simulink model "OFDM_Rx_HW"  (R2020a)
settings: Solver=FixedStepDiscrete  StartTime=0.0  StopTime=inf  RelTol=1e-3
InitFcn:
  | % Set parameters
  | fs = 20e6;
  | fclk = 240e6;
  | ssr = 2;
  | fdc = fclk*ssr*8;
  | 
  | % Load libraries
  | addpath('./lib');
  | 
  | % Load all required variables
  | load('variables/read_addr_data');
  | load('variables/read_addr_cp');
  | load('variables/read_addr_pream');
  | load('variables/read_addr_rx');
  | load('variables/pilot');
  | load('variables/sc_index');
  | load('variables/LTSfreq');
  | load('variables/STSfreq');
  | load('variables/LTSread');
  | load('variables/STSread');
  | 
  | run ./scripts/rfgen;
undefined symbols (not defined in the file): LTSfreq, pilot, read_addr_rx, sc_index
libraries: simulink x36, hdlsllib x30, dsphdlmathfun x3, dspsigops x2, dsphdlxfrm x1, dsphdlsigops x1
(part 1 of 3)
settings Model: DataTypeOverride=Off  Creator=njb13206  LastModifiedBy=andy
settings OptimizationCC: BlockReduction=off  ConditionallyExecuteInputs=off  DefaultParameterBehavior=Inlined
settings DebuggingCC: AlgebraicLoopMsg=error  SingleTaskRateTransMsg=error  IntegerOverflowMsg=none  ParameterPrecisionLossMsg=none  IntegerSaturationMsg=none
settings HardwareCC: ProdBitPerPointer=32  ProdBitPerSizeT=32  ProdBitPerPtrDiffT=32  ProdLargestAtomicFloat=None  ProdIntDivRoundTo=Undefined  ProdEndianess=Unspecified  ProdWordSize=32  ProdHWDeviceType=ASIC/FPGA->ASIC/FPGA  TargetBitPerLong=64  TargetBitPerPointer=64  TargetBitPerSizeT=64  TargetBitPerPtrDiffT=64  TargetLongLongMode=on  TargetIntDivRoundTo=Zero  TargetEndianess=LittleEndian  TargetWordSize=64  TargetHWDeviceType=Custom Processor->MATLAB Host Computer  ProdEqTarget=off

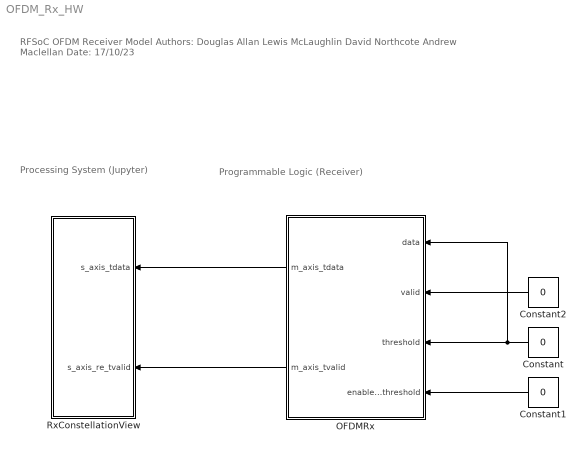
== system OFDM_Rx_HW ==
  note: Processing System (Jupyter)
  note: RFSoC OFDM Receiver Model
      | Authors: Douglas Allan
      | Lewis McLaughlin
      | David Northcote
      | Andrew Maclellan
      | Date: 17/10/23
  note: Programmable Logic (Receiver)
  Constant : Constant  Value=0  OutDataTypeStr=uint32  SampleTime=-1
  Constant1 : Constant  Value=0  OutDataTypeStr=uint32  SampleTime=-1
  Constant2 : Constant  Value=0  OutDataTypeStr=boolean  SampleTime=-1
  OFDMRx : Subsystem  TreatAsAtomicUnit=on
  RxConstellationView : Subsystem
  wires:
  OFDMRx/1(m_axis_tdata) -> RxConstellationView/1(s_axis_tdata)
  OFDMRx/2(m_axis_tvalid) -> RxConstellationView/2(s_axis_re_tvalid)
  Constant1/1 -> OFDMRx/4(enable_threshold)
  Constant/1 -> OFDMRx/3(threshold), OFDMRx/1(data)
  Constant2/1 -> OFDMRx/2(valid)

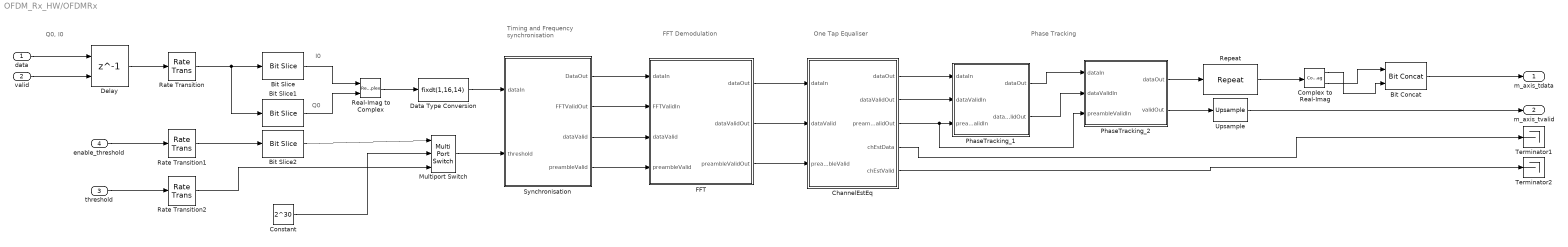
== system OFDM_Rx_HW/OFDMRx ==
  note: Phase Tracking
  note: One Tap Equaliser
  note: FFT Demodulation
  note: Timing and Frequency
      | synchronisation
  note: Q0, I0
  note: I0
  note: Q0
  data : Inport
  valid : Inport  Port=2
  threshold : Inport  Port=3
  enable_threshold : Inport  Port=4
  Bit Concat : hdlsllib/Logic and Bit Operations/Bit Concat  numInputs=2
  Bit Slice : hdlsllib/Logic and Bit Operations/Bit Slice  lidx=15  ridx=0
      settings: SourceProductBaseCode=SL
  Bit Slice1 : hdlsllib/Logic and Bit Operations/Bit Slice  lidx=31  ridx=16
      settings: SourceProductBaseCode=SL
  Bit Slice2 : hdlsllib/Logic and Bit Operations/Bit Slice  lidx=0  ridx=0
      settings: SourceProductBaseCode=SL
  ChannelEstEq : Subsystem
  Complex to Real-Imag : ComplexToRealImag
  Constant : Constant  Value=2^30  OutDataTypeStr=uint32  SampleTime=-1
  Data Type Conversion : DataTypeConversion  OutDataTypeStr=fixdt(1,16,14)  ConvertRealWorld=Stored Integer (SI)
  Delay : Delay  DelayLength=1  ShowEnablePort=on
      settings: InputPortMap=u0,e6
  FFT : Subsystem
  Multiport Switch : MultiPortSwitch  DataPortOrder=Zero-based contiguous  Inputs=2  zeroidx=on
  PhaseTracking_1 : Subsystem
  PhaseTracking_2 : Subsystem
  Rate Transition : RateTransition  OutPortSampleTime=1/fs
  Rate Transition1 : RateTransition  OutPortSampleTime=1/fs
  Rate Transition2 : RateTransition  OutPortSampleTime=1/fs
  Real-Imag to Complex : RealImagToComplex
  Repeat : dspsigops/Repeat  N=12  InputProcessing=Columns as channels (frame based)  RateOptions=Allow multirate processing  ic=0  mode=Unused parameter value
  Synchronisation : Subsystem
  Terminator1 : Terminator
  Terminator2 : Terminator
  Upsample : dspsigops/Upsample  N=12  phase=5  RateOptions=Allow multirate processing  ic=0  mode=Unused parameter value
  m_axis_tdata : Outport  VectorParamsAs1DForOutWhenUnconnected=off
  m_axis_tvalid : Outport  Port=2  VectorParamsAs1DForOutWhenUnconnected=off
  wires:
  valid/1 -> Delay/2
  Bit Slice1/1 -> Real-Imag to Complex/2
  Bit Slice/1 -> Real-Imag to Complex/1
  Complex to Real-Imag/1 -> Bit Concat/2
  Complex to Real-Imag/2 -> Bit Concat/1
  Repeat/1 -> Complex to Real-Imag/1
  PhaseTracking_2/2(validOut) -> Upsample/1
  PhaseTracking_2/1(dataOut) -> Repeat/1
  Data Type Conversion/1 -> Synchronisation/1(dataIn)
  Real-Imag to Complex/1 -> Data Type Conversion/1
  FFT/1(dataOut) -> ChannelEstEq/1(dataIn)
  FFT/3(preambleValidOut) -> ChannelEstEq/3(preambleValid)
  FFT/2(dataValidOut) -> ChannelEstEq/2(dataValid)
  Synchronisation/1(DataOut) -> FFT/1(dataIn)
  Synchronisation/2(FFTValidOut) -> FFT/2(FFTValidIn)
  Synchronisation/3(dataValid) -> FFT/3(dataValid)
  Synchronisation/4(preambleValid) -> FFT/4(preambleValid)
  ChannelEstEq/1(dataOut) -> PhaseTracking_1/1(dataIn)
  ChannelEstEq/2(dataValidOut) -> PhaseTracking_1/2(dataValidIn)
  PhaseTracking_1/1(dataOut) -> PhaseTracking_2/1(dataIn)
  PhaseTracking_1/2(dataValidOut) -> PhaseTracking_2/2(dataValidIn)
  ChannelEstEq/5(chEstValid) -> Terminator2/1
  ChannelEstEq/4(chEstData) -> Terminator1/1
  Multiport Switch/1 -> Synchronisation/2(threshold)
  threshold/1 -> Rate Transition2/1
  Constant/1 -> Multiport Switch/2
  enable_threshold/1 -> Rate Transition1/1
  Bit Concat/1 -> m_axis_tdata/1
  Upsample/1 -> m_axis_tvalid/1
  Bit Slice2/1 -> Multiport Switch/1
  Rate Transition/1 -> Bit Slice/1, Bit Slice1/1
  Rate Transition1/1 -> Bit Slice2/1
  Rate Transition2/1 -> Multiport Switch/3
  Delay/1 -> Rate Transition/1
  data/1 -> Delay/1
  ChannelEstEq/3(preambleValidOut) -> PhaseTracking_2/3(preambleValidIn), PhaseTracking_1/3(preambleValidIn)

== system OFDM_Rx_HW/RxConstellationView ==
  s_axis_tdata : Inport
  s_axis_re_tvalid : Inport  Port=2
  Bit Slice : hdlsllib/Logic and Bit Operations/Bit Slice  lidx=15  ridx=0
      settings: SourceProductBaseCode=SL
  Bit Slice1 : hdlsllib/Logic and Bit Operations/Bit Slice  lidx=31  ridx=16
      settings: SourceProductBaseCode=SL
  Constant : Constant  Value=NaN + 1i*NaN  OutDataTypeStr=double  SampleTime=-1
  Constellation Diagram : ConstellationDiagram
  Data Type Conversion : DataTypeConversion  OutDataTypeStr=fixdt(1,16,14)  ConvertRealWorld=Stored Integer (SI)
  Real-Imag to Complex : RealImagToComplex
  Switch : Switch  Criteria=u2 ~= 0
  wires:
  Switch/1 -> Constellation Diagram/1
  Constant/1 -> Switch/3
  s_axis_re_tvalid/1 -> Switch/2
  Real-Imag to Complex/1 -> Data Type Conversion/1
  Bit Slice/1 -> Real-Imag to Complex/1
  s_axis_tdata/1 -> Bit Slice1/1, Bit Slice/1
  Bit Slice1/1 -> Real-Imag to Complex/2
  Data Type Conversion/1 -> Switch/1

== system OFDM_Rx_HW/OFDMRx/ChannelEstEq ==
  dataIn : Inport
  dataValid : Inport  Port=2
  preambleValid : Inport  Port=3
  Bit Concat1 : hdlsllib/Logic and Bit Operations/Bit Concat  numInputs=2
  ChannelEstimate : Subsystem
  Complex to Real-Imag1 : ComplexToRealImag
  Data Type Conversion1 : DataTypeConversion  OutDataTypeStr=fixdt(1,16,14)
  Data Type Conversion3 : DataTypeConversion  OutDataTypeStr=uint16  ConvertRealWorld=Stored Integer (SI)
  Data Type Conversion4 : DataTypeConversion  OutDataTypeStr=uint16  ConvertRealWorld=Stored Integer (SI)
  Delay : Delay  DelayLength=6
  Delay1 : Delay  DelayLength=6
  Delay2 : Delay  DelayLength=5
  Equalise : Subsystem
  dataOut : Outport  VectorParamsAs1DForOutWhenUnconnected=off
  dataValidOut : Outport  Port=2  VectorParamsAs1DForOutWhenUnconnected=off
  preambleValidOut : Outport  Port=3  VectorParamsAs1DForOutWhenUnconnected=off
  chEstData : Outport  Port=4  VectorParamsAs1DForOutWhenUnconnected=off
  chEstValid : Outport  Port=5  VectorParamsAs1DForOutWhenUnconnected=off
  wires:
  ChannelEstimate/1(chEstOut) -> Equalise/2(chEstIn), Data Type Conversion1/1
  Delay/1 -> Equalise/1(dataInEq)
  dataIn/1 -> ChannelEstimate/1(dataIn), Delay/1
  preambleValid/1 -> Delay1/1, ChannelEstimate/2(preambleValid)
  dataValid/1 -> ChannelEstimate/3(dataValidIn)
  Equalise/1(dataOutEq) -> dataOut/1
  Equalise/2(dataValidOut) -> dataValidOut/1
  ChannelEstimate/2(dataValidOut) -> chEstValid/1, Equalise/3(dataValidIn)
  Data Type Conversion4/1 -> Bit Concat1/1
  Bit Concat1/1 -> chEstData/1
  Data Type Conversion3/1 -> Bit Concat1/2
  Complex to Real-Imag1/2 -> Data Type Conversion4/1
  Complex to Real-Imag1/1 -> Data Type Conversion3/1
  Data Type Conversion1/1 -> Complex to Real-Imag1/1
  Delay1/1 -> Delay2/1
  Delay2/1 -> preambleValidOut/1

== system OFDM_Rx_HW/OFDMRx/FFT ==
  dataIn : Inport
  FFTValidIn : Inport  Port=2
  dataValid : Inport  Port=3
  preambleValid : Inport  Port=4
  Delay1 : Delay  DelayLength=173
  Delay2 : Delay  DelayLength=173
  FFT HDL Optimized : dsphdlxfrm/FFT HDL Optimized  FFTLength=64  Architecture=Streaming Radix 2^2  ComplexMultiplication=Use 4 multipliers and 2 adders  BitReversedOutput=off  BitReversedInput=off  Normalize=off  SimulateUsing=Code generation  RoundingMethod=Floor  ResetInputPort=off  StartOutputPort=off  EndOutputPort=off
      settings: SourceProductBaseCode=DS
  Terminator : Terminator
  dataOut : Outport  VectorParamsAs1DForOutWhenUnconnected=off
  dataValidOut : Outport  Port=2  VectorParamsAs1DForOutWhenUnconnected=off
  preambleValidOut : Outport  Port=3  VectorParamsAs1DForOutWhenUnconnected=off
  wires:
  FFTValidIn/1 -> FFT HDL Optimized/2
  dataIn/1 -> FFT HDL Optimized/1
  Delay2/1 -> dataValidOut/1
  Delay1/1 -> preambleValidOut/1
  FFT HDL Optimized/1 -> dataOut/1
  FFT HDL Optimized/2 -> Terminator/1
  dataValid/1 -> Delay2/1
  preambleValid/1 -> Delay1/1

== system OFDM_Rx_HW/OFDMRx/PhaseTracking_1 ==
  note: Phase Tracking Stage 1: Track linear phase error which occurs due to sampling phase/frequency offsets. The implemented algorithm
      | estimates the gradient of the linear phase error using pilot sub-carriers.
  dataIn : Inport
  dataValidIn : Inport  Port=2
  preambleValidIn : Inport  Port=3
  CordicRotate : Subsystem
  DataArrange : Subsystem
  "GradientEstimate " : Subsystem
  PhaseErrorEst : Subsystem
  PilotCtrlGen : Subsystem
  dataOut : Outport
  dataValidOut : Outport  Port=2
  wires:
  CordicRotate/2(dataValidOut) -> dataValidOut/1
  PhaseErrorEst/3(dataValidOut) -> CordicRotate/3(dataValidIn)
  PhaseErrorEst/2(PhaseOut) -> CordicRotate/2(PhaseInRotate)
  PhaseErrorEst/1(dataOut) -> CordicRotate/1(DataInRotate)
  "GradientEstimate "/1(dataOut) -> PhaseErrorEst/1(dataIn)
  "GradientEstimate "/2(gradientOut) -> PhaseErrorEst/2(gradientIn)
  "GradientEstimate "/3(dataValidOut) -> PhaseErrorEst/3(dataValidIn)
  CordicRotate/1("DataOutRotate  ") -> dataOut/1
  dataIn/1 -> DataArrange/1(dataIn)
  dataValidIn/1 -> DataArrange/2(dataValidIn)
  DataArrange/1(dataOut) -> PilotCtrlGen/1(dataIn)
  DataArrange/2(dataValidOut) -> PilotCtrlGen/2(validIn)
  PilotCtrlGen/1(dataOut) -> "GradientEstimate "/1(dataIn)
  PilotCtrlGen/2(pilotOut) -> "GradientEstimate "/2(pilotIn)
  PilotCtrlGen/3(pilotEnd) -> "GradientEstimate "/3(PilotEnd)
  PilotCtrlGen/4(dataValid) -> "GradientEstimate "/4(dataValid)
  DataArrange/3(frameDetOut) -> PilotCtrlGen/3(preambleValidIn)
  preambleValidIn/1 -> DataArrange/3(preambleValidIn)

== system OFDM_Rx_HW/OFDMRx/PhaseTracking_2 ==
  note: Phase Tracking Stage 2:  Track Common Phase Error (CPE) from symbol to symbol.
      | CPE is caused by residual frequency offset and phase noise effects.
  dataIn : Inport
  dataValidIn : Inport  Port=2
  preambleValidIn : Inport  Port=3
  CordicRotate : Subsystem
  PhaseEst : Subsystem
  PilotCtrlGen : Subsystem
  dataOut : Outport  VectorParamsAs1DForOutWhenUnconnected=off
  validOut : Outport  Port=2  VectorParamsAs1DForOutWhenUnconnected=off
  wires:
  PilotCtrlGen/1(dataOut) -> PhaseEst/1(dataIn)
  PilotCtrlGen/2(pilotOut) -> PhaseEst/2(PilotIn)
  PilotCtrlGen/3(PilotEnd) -> PhaseEst/3(pilotEnd)
  PilotCtrlGen/4(dataValid) -> PhaseEst/4(dataValid)
  PhaseEst/1(dataOut) -> CordicRotate/1(DataIn)
  PhaseEst/2(phaseOut) -> CordicRotate/2(PhaseIn)
  PhaseEst/3(validOut) -> CordicRotate/3(validIn)
  CordicRotate/1("DataOut  ") -> dataOut/1
  CordicRotate/2(validOut) -> validOut/1
  dataIn/1 -> PilotCtrlGen/1(dataIn)
  dataValidIn/1 -> PilotCtrlGen/2(ValidIn)
  preambleValidIn/1 -> PilotCtrlGen/3(preambleValidIn)

== system OFDM_Rx_HW/OFDMRx/Synchronisation ==
  dataIn : Inport
  threshold : Inport  Port=2
  CoarseFreqCorr : Subsystem
  ControlSigGen : Subsystem
  Delay : Subsystem
  Delay1 : Delay  DelayLength=22  InputProcessing=Columns as channels (frame based)
  Delay2 : Delay  InputProcessing=Columns as channels (frame based)
  Delay4 : Delay  DelayLength=1  InputProcessing=Columns as channels (frame based)
  FrameDetect : Subsystem
  "SchmidlCoxMetric " : Subsystem
  DataOut : Outport  VectorParamsAs1DForOutWhenUnconnected=off
  FFTValidOut : Outport  Port=2  VectorParamsAs1DForOutWhenUnconnected=off
  dataValid : Outport  Port=3  VectorParamsAs1DForOutWhenUnconnected=off
  preambleValid : Outport  Port=4  VectorParamsAs1DForOutWhenUnconnected=off
  wires:
  dataIn/1 -> "SchmidlCoxMetric "/1(dataIn), Delay1/1
  ControlSigGen/1(FFTValid) -> FFTValidOut/1
  ControlSigGen/2(dataValid) -> dataValid/1
  ControlSigGen/3(preambleValid) -> preambleValid/1  "preamble"
  Delay1/1 -> Delay2/1
  "SchmidlCoxMetric "/1(left) -> FrameDetect/1(leftIn)
  "SchmidlCoxMetric "/2(right) -> FrameDetect/2(rightIn)
  "SchmidlCoxMetric "/3(phase) -> FrameDetect/3(phaseIn)
  FrameDetect/2(phaseOut) -> CoarseFreqCorr/3(phaseIn)
  Delay2/1 -> CoarseFreqCorr/1(dataIn)
  FrameDetect/1(frameDet) -> CoarseFreqCorr/2(frameDet)
  Delay4/1 -> DataOut/1
  CoarseFreqCorr/2(frameDetOut) -> Delay/2(strobe)
  CoarseFreqCorr/1(dataOut) -> Delay/1(data)
  Delay/2(strobeOut) -> ControlSigGen/1(validIn)
  Delay/1(dataOut) -> Delay4/1
  threshold/1 -> "SchmidlCoxMetric "/2(threshold)

== system OFDM_Rx_HW/OFDMRx/ChannelEstEq/ChannelEstimate ==
  note: Note the preamble symbols do not pass this point.
  note: Write averaged channel estimate to RAM and read out when data is valid
      | for equalisation of successive OFDM symbols.
  note: Get and store the channel estimate using the two
      | repetitions of the L-LTF
  dataIn : Inport
  preambleValid : Inport  Port=2
  dataValidIn : Inport  Port=3
  ChanEst : Subsystem
  Delay : Delay  DelayLength=5
  Delay1 : Delay  DelayLength=5
  Delay2 : Delay  DelayLength=1
  Dual Port RAM1 : hdlsllib/HDL RAMs/Dual Port RAM  ram_size=6
      settings: SourceProductBaseCode=SL
  HDL Counter3 : hdlsllib/Sources/HDL Counter  CountType=Count limited  CountInit=0  CountStep=1  CountMax=63  CountFromType=Initial value  CountFrom=0  CountResetPort=off  CountLoadPort=off  CountEnbPort=on  CountDirPort=off  CountDataType=Unsigned  CountWordLen=6  CountFracLen=0  CountSampTime=1
  Terminator : Terminator
  WriteEnbAddrGen : Subsystem
  chEstOut : Outport  VectorParamsAs1DForOutWhenUnconnected=off
  dataValidOut : Outport  Port=2  VectorParamsAs1DForOutWhenUnconnected=off
  wires:
  HDL Counter3/1 -> Dual Port RAM1/4
  Dual Port RAM1/2 -> chEstOut/1
  Delay2/1 -> dataValidOut/1
  preambleValid/1 -> ChanEst/2(PreambValidIn), Delay/1
  dataIn/1 -> ChanEst/1(ChanEstIn)
  ChanEst/1(ChEstOut) -> Dual Port RAM1/1
  dataValidIn/1 -> Delay1/1
  Delay1/1 -> HDL Counter3/1, Delay2/1
  Delay/1 -> WriteEnbAddrGen/1(In1)
  WriteEnbAddrGen/1(Out1) -> Dual Port RAM1/2
  WriteEnbAddrGen/2(Out2) -> Dual Port RAM1/3
  Dual Port RAM1/1 -> Terminator/1

== system OFDM_Rx_HW/OFDMRx/ChannelEstEq/Equalise ==
  note: Perform a complex division to obtain equalised data symbols.
  dataInEq : Inport
  chEstIn : Inport  Port=2
  dataValidIn : Inport  Port=3
  Abs2 : Subsystem
  Complex Mult : Subsystem
  Delay1 : Delay
  Delay8 : Delay  DelayLength=3
  Divide : Subsystem
  dataOutEq : Outport  VectorParamsAs1DForOutWhenUnconnected=off
  dataValidOut : Outport  Port=2  VectorParamsAs1DForOutWhenUnconnected=off
  wires:
  dataValidIn/1 -> Delay8/1
  chEstIn/1 -> Abs2/1(ChEstIn), Complex Mult/2(In2)
  dataInEq/1 -> Complex Mult/1(In1)
  Complex Mult/1(Out1) -> Divide/1(In1)
  Abs2/1(Out1) -> Divide/2(In2)
  Delay8/1 -> Delay1/1
  Delay1/1 -> dataValidOut/1
  Divide/1(dataOutEq) -> dataOutEq/1

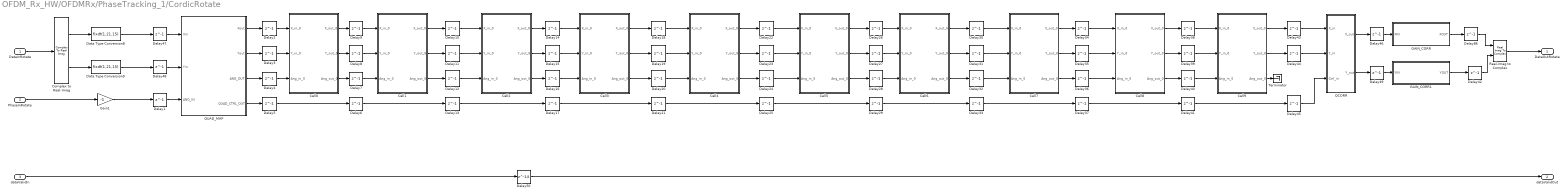
== system OFDM_Rx_HW/OFDMRx/PhaseTracking_1/CordicRotate ==
  DataInRotate : Inport
  PhaseInRotate : Inport  Port=2
  dataValidIn : Inport  Port=3
  Cell0 : Subsystem
  Cell1 : Subsystem
  Cell2 : Subsystem
  Cell3 : Subsystem
  Cell4 : Subsystem
  Cell5 : Subsystem
  Cell6 : Subsystem
  Cell7 : Subsystem
  Cell8 : Subsystem
  Cell9 : Subsystem
  Complex to Real-Imag : ComplexToRealImag
  Data Type Conversion8 : DataTypeConversion  OutDataTypeStr=fixdt(1,21,15)
  Data Type Conversion9 : DataTypeConversion  OutDataTypeStr=fixdt(1,21,15)
  Delay{1..49,86} (50 alike) : Delay  DelayLength=1
  Delay50 : Delay  DelayLength=14
  GAIN_CORR : Subsystem
  GAIN_CORR1 : Subsystem
  Gain1 : Gain  Gain=-1  OutDataTypeStr=fixdt(1,23,20)
  QCORR : Subsystem
  QUAD_MAP : Subsystem
  Real-Imag to Complex : RealImagToComplex
  Terminator : Terminator
  "DataOutRotate  " : Outport  VectorParamsAs1DForOutWhenUnconnected=off
  dataValidOut : Outport  Port=2  VectorParamsAs1DForOutWhenUnconnected=off
  wires:
  Delay50/1 -> dataValidOut/1
  dataValidIn/1 -> Delay50/1
  Gain1/1 -> Delay1/1
  PhaseInRotate/1 -> Gain1/1
  QCORR/1(X_out) -> Delay46/1
  Data Type Conversion9/1 -> Delay48/1
  Data Type Conversion8/1 -> Delay47/1
  Delay45/1 -> QCORR/3(Ctrl_in)
  Delay4/1 -> Cell0/3(Ang_in_0)
  Delay1/1 -> QUAD_MAP/3(ANG_IN)
  QCORR/2(Y_out) -> Delay49/1
  Delay49/1 -> GAIN_CORR1/1(YIN)
  Delay46/1 -> GAIN_CORR/1(XIN)
  Delay44/1 -> QCORR/2(Y_in)
  Delay43/1 -> QCORR/1(X_in)
  Cell9/2(Y_out_0) -> Delay44/1
  Cell9/1(X_out_0) -> Delay43/1
  Delay41/1 -> Delay45/1
  Cell9/3(Ang_out_0) -> Terminator/1
  GAIN_CORR1/1(YOUT) -> Delay42/1
  Cell8/1(X_out_0) -> Delay38/1
  Cell8/2(Y_out_0) -> Delay39/1
  Cell8/3(Ang_out_0) -> Delay40/1
  Delay37/1 -> Delay41/1
  Delay38/1 -> Cell9/1(X_in_0)
  Delay39/1 -> Cell9/2(Y_in_0)
  Delay40/1 -> Cell9/3(Ang_in_0)
  Delay36/1 -> Cell8/3(Ang_in_0)
  Delay35/1 -> Cell8/2(Y_in_0)
  Delay34/1 -> Cell8/1(X_in_0)
  Delay33/1 -> Delay37/1
  Cell7/3(Ang_out_0) -> Delay36/1
  Cell7/2(Y_out_0) -> Delay35/1
  Cell7/1(X_out_0) -> Delay34/1
  Cell6/1(X_out_0) -> Delay30/1
  Cell6/2(Y_out_0) -> Delay31/1
  Cell6/3(Ang_out_0) -> Delay32/1
  Delay29/1 -> Delay33/1
  Delay30/1 -> Cell7/1(X_in_0)
  Delay31/1 -> Cell7/2(Y_in_0)
  Delay32/1 -> Cell7/3(Ang_in_0)
  Delay28/1 -> Cell6/3(Ang_in_0)
  Delay27/1 -> Cell6/2(Y_in_0)
  Delay26/1 -> Cell6/1(X_in_0)
  Delay25/1 -> Delay29/1
  Cell5/3(Ang_out_0) -> Delay28/1
  Cell5/2(Y_out_0) -> Delay27/1
  Cell5/1(X_out_0) -> Delay26/1
  Cell4/1(X_out_0) -> Delay22/1
  Cell4/2(Y_out_0) -> Delay23/1
  Cell4/3(Ang_out_0) -> Delay24/1
  Delay21/1 -> Delay25/1
  Delay22/1 -> Cell5/1(X_in_0)
  Delay23/1 -> Cell5/2(Y_in_0)
  Delay24/1 -> Cell5/3(Ang_in_0)
  Delay20/1 -> Cell4/3(Ang_in_0)
  Delay19/1 -> Cell4/2(Y_in_0)
  Delay18/1 -> Cell4/1(X_in_0)
  Delay17/1 -> Delay21/1
  Cell3/3(Ang_out_0) -> Delay20/1
  Cell3/2(Y_out_0) -> Delay19/1
  Cell3/1(X_out_0) -> Delay18/1
  Cell2/1(X_out_0) -> Delay14/1
  Cell2/2(Y_out_0) -> Delay15/1
  Cell2/3(Ang_out_0) -> Delay16/1
  Delay13/1 -> Delay17/1
  Delay14/1 -> Cell3/1(X_in_0)
  Delay15/1 -> Cell3/2(Y_in_0)
  Delay16/1 -> Cell3/3(Ang_in_0)
  Delay12/1 -> Cell2/3(Ang_in_0)
  Delay11/1 -> Cell2/2(Y_in_0)
  Delay10/1 -> Cell2/1(X_in_0)
  Delay6/1 -> Delay13/1
  Cell1/3(Ang_out_0) -> Delay12/1
  Cell1/2(Y_out_0) -> Delay11/1
  Cell1/1(X_out_0) -> Delay10/1
  Delay9/1 -> Cell1/1(X_in_0)
  Delay8/1 -> Cell1/2(Y_in_0)
  Delay7/1 -> Cell1/3(Ang_in_0)
  Delay5/1 -> Delay6/1
  Cell0/3(Ang_out_0) -> Delay7/1
  Cell0/2(Y_out_0) -> Delay8/1
  Cell0/1(X_out_0) -> Delay9/1
  QUAD_MAP/4(QUAD_CTRL_OUT) -> Delay5/1
  Delay3/1 -> Cell0/2(Y_in_0)
  Delay2/1 -> Cell0/1(X_in_0)
  QUAD_MAP/3(ANG_OUT) -> Delay4/1
  QUAD_MAP/2(Yout) -> Delay3/1
  QUAD_MAP/1(Xout) -> Delay2/1
  Delay47/1 -> QUAD_MAP/1(Xin)
  Delay48/1 -> QUAD_MAP/2(Yin)
  GAIN_CORR/1(XOUT) -> Delay86/1
  Complex to Real-Imag/2 -> Data Type Conversion9/1
  DataInRotate/1 -> Complex to Real-Imag/1
  Complex to Real-Imag/1 -> Data Type Conversion8/1
  Delay86/1 -> Real-Imag to Complex/1
  Delay42/1 -> Real-Imag to Complex/2
  Real-Imag to Complex/1 -> "DataOutRotate  "/1

== system OFDM_Rx_HW/OFDMRx/PhaseTracking_1/DataArrange ==
  note: Re-arrange data symbols
  dataIn : Inport
  dataValidIn : Inport  Port=2
  preambleValidIn : Inport  Port=3
  Delay : Delay  DelayLength=64  InitialCondition=0  UseCircularBuffer=on
  Delay1 : Delay  DelayLength=65
  Delay3 : Delay  DelayLength=1  InitialCondition=0  UseCircularBuffer=on
  Dual Port RAM : hdlsllib/HDL RAMs/Dual Port RAM  ram_size=7
      settings: SourceProductBaseCode=SL
  HDL Counter : hdlsllib/Sources/HDL Counter  CountType=Count limited  CountInit=0  CountStep=1  CountMax=127  CountFromType=Initial value  CountFrom=0  CountResetPort=off  CountLoadPort=off  CountEnbPort=on  CountDirPort=off  CountDataType=Unsigned  CountWordLen=7  CountFracLen=0  CountSampTime=1
  HDL Counter1 : hdlsllib/Sources/HDL Counter  CountType=Count limited  CountInit=0  CountStep=1  CountMax=127  CountFromType=Initial value  CountFrom=0  CountResetPort=off  CountLoadPort=off  CountEnbPort=on  CountDirPort=off  CountDataType=Unsigned  CountWordLen=7  CountFracLen=0  CountSampTime=1
  READ_ADDRESS : Lookup_n-D  NumberOfTableDimensions=1  LookupTableObject=''  BreakpointsForDimension1=[0:127]  BreakpointsForDimension1FirstPoint=10  BreakpointsForDimension2FirstPoint=10  BreakpointsForDimension1Spacing=12  BreakpointsForDimension2Spacing=12  IndexSearchMethod=Evenly spaced points  Table=read_addr_rx  TableDataTypeStr=fixdt(0,7,0)  InterpMethod=Flat  DiagnosticForOutOfRangeInput=Error  InternalRulePriority=Speed  OutDataTypeStr=fixdt(0,7,0)  RndMeth=Simplest  InputSameDT=on
  READ_CTRL : Subsystem
  Terminator : Terminator
  dataValidGen : Subsystem
  dataOut : Outport  VectorParamsAs1DForOutWhenUnconnected=off
  dataValidOut : Outport  Port=2  VectorParamsAs1DForOutWhenUnconnected=off
  frameDetOut : Outport  Port=3  VectorParamsAs1DForOutWhenUnconnected=off
  wires:
  Dual Port RAM/1 -> Terminator/1
  dataValidIn/1 -> Delay/1, HDL Counter1/1, Dual Port RAM/3
  HDL Counter/1 -> READ_ADDRESS/1
  Dual Port RAM/2 -> dataOut/1
  dataIn/1 -> Dual Port RAM/1
  HDL Counter1/1 -> Dual Port RAM/2
  Delay/1 -> HDL Counter/1, Delay3/1, READ_CTRL/2(In2)
  READ_CTRL/1(Out1) -> Dual Port RAM/4
  READ_ADDRESS/1 -> READ_CTRL/1(In1)
  Delay3/1 -> dataValidGen/1(enb)
  dataValidGen/1(dataValidOut) -> dataValidOut/1
  Delay1/1 -> frameDetOut/1
  preambleValidIn/1 -> Delay1/1

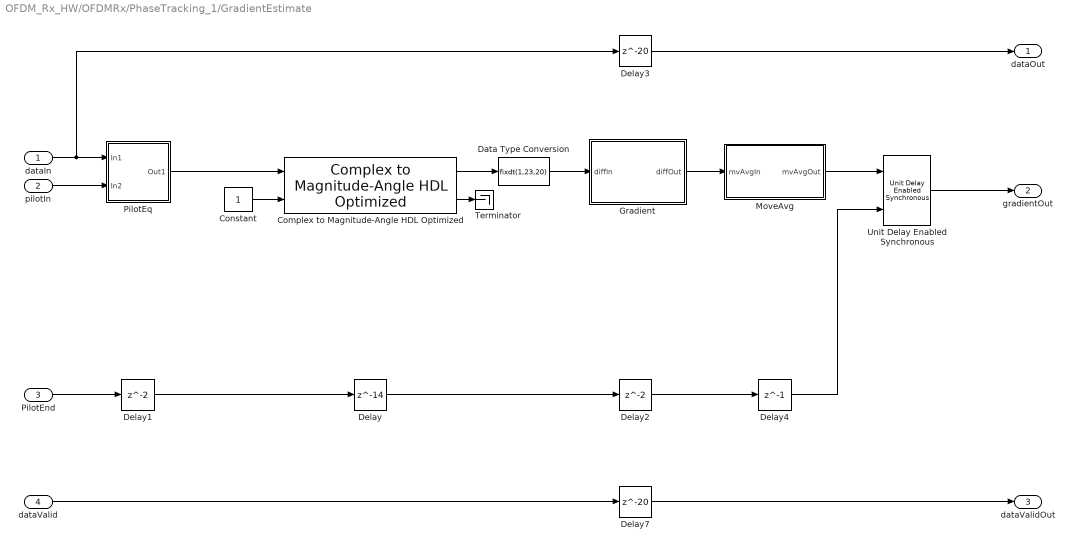
== system OFDM_Rx_HW/OFDMRx/PhaseTracking_1/GradientEstimate  ==
  dataIn : Inport
  pilotIn : Inport  Port=2
  PilotEnd : Inport  Port=3
  dataValid : Inport  Port=4
  Complex to Magnitude-Angle HDL Optimized : dsphdlmathfun/Complex to Magnitude-Angle HDL Optimized  NumIterationsSource=Property  NumIterations=10  OutputFormat=Angle  AngleFormat=Radians  ScaleOutput=off  SimulateUsing=Code generation
      settings: SourceProductBaseCode=DS
  Constant : Constant  OutDataTypeStr=boolean  SampleTime=1/fs
  Data Type Conversion : DataTypeConversion  OutDataTypeStr=fixdt(1,23,20)
  Delay : Delay  DelayLength=14
  Delay1 : Delay
  Delay2 : Delay
  Delay3 : Delay  DelayLength=20
  Delay4 : Delay  DelayLength=1
  Delay7 : Delay  DelayLength=20
  Gradient : Subsystem
  MoveAvg : Subsystem
  PilotEq : Subsystem
  Terminator : Terminator
  Unit Delay Enabled Synchronous : hdlsllib/Discrete/Unit Delay Enabled Synchronous  InitialCondition=0.0  SampleTime=-1
      settings: SourceProductBaseCode=SL
  dataOut : Outport  VectorParamsAs1DForOutWhenUnconnected=off
  gradientOut : Outport  Port=2  VectorParamsAs1DForOutWhenUnconnected=off
  dataValidOut : Outport  Port=3  VectorParamsAs1DForOutWhenUnconnected=off
  wires:
  Delay2/1 -> Delay4/1
  Data Type Conversion/1 -> Gradient/1(diffIn)
  Complex to Magnitude-Angle HDL Optimized/2 -> Terminator/1
  Constant/1 -> Complex to Magnitude-Angle HDL Optimized/2
  Complex to Magnitude-Angle HDL Optimized/1 -> Data Type Conversion/1
  Delay7/1 -> dataValidOut/1
  Unit Delay Enabled Synchronous/1 -> gradientOut/1
  Delay3/1 -> dataOut/1
  MoveAvg/1(mvAvgOut) -> Unit Delay Enabled Synchronous/1
  Delay1/1 -> Delay/1
  PilotEq/1(Out1) -> Complex to Magnitude-Angle HDL Optimized/1
  pilotIn/1 -> PilotEq/2(In2)
  dataIn/1 -> PilotEq/1(In1), Delay3/1
  Gradient/1(diffOut) -> MoveAvg/1(mvAvgIn)
  dataValid/1 -> Delay7/1
  PilotEnd/1 -> Delay1/1
  Delay/1 -> Delay2/1
  Delay4/1 -> Unit Delay Enabled Synchronous/2

== system OFDM_Rx_HW/OFDMRx/PhaseTracking_1/PhaseErrorEst ==
  dataIn : Inport
  gradientIn : Inport  Port=2
  dataValidIn : Inport  Port=3
  Delay{2..8} (7 alike) : Delay  DelayLength=1
  HDL Counter : hdlsllib/Sources/HDL Counter  CountType=Count limited  CountInit=0  CountStep=1  CountMax=51  CountFromType=Initial value  CountFrom=0  CountResetPort=on  CountLoadPort=off  CountEnbPort=on  CountDirPort=off  CountDataType=Unsigned  CountWordLen=6  CountFracLen=0  CountSampTime=1
  LUT : Lookup_n-D  NumberOfTableDimensions=1  BreakpointsForDimension1=0:51  IndexSearchMethod=Evenly spaced points  Table=sc_index  TableDataTypeStr=fixdt(1,6,0)  InterpMethod=Flat  ExtrapMethod=Clip  DiagnosticForOutOfRangeInput=Error  UseLastTableValue=on  InternalRulePriority=Speed  OutDataTypeStr=fixdt(1,6,0)  RndMeth=Simplest  InputSameDT=on
  NOT : Logic  Operator=NOT  IconShape=distinctive  AllPortsSameDT=off  OutDataTypeStr=boolean
  Product : Product  OutDataTypeStr=fixdt(1,23,20)
  dataOut : Outport  VectorParamsAs1DForOutWhenUnconnected=off
  PhaseOut : Outport  Port=2  VectorParamsAs1DForOutWhenUnconnected=off
  dataValidOut : Outport  Port=3  VectorParamsAs1DForOutWhenUnconnected=off
  wires:
  Delay8/1 -> dataValidOut/1
  Delay4/1 -> Delay8/1
  Delay7/1 -> PhaseOut/1
  Product/1 -> Delay7/1
  Delay6/1 -> dataOut/1
  Delay2/1 -> Delay6/1
  Delay5/1 -> Product/2
  Delay3/1 -> Product/1
  HDL Counter/1 -> LUT/1
  NOT/1 -> HDL Counter/1
  LUT/1 -> Delay5/1
  gradientIn/1 -> Delay3/1
  dataIn/1 -> Delay2/1
  dataValidIn/1 -> HDL Counter/2, Delay4/1, NOT/1

== system OFDM_Rx_HW/OFDMRx/PhaseTracking_1/PilotCtrlGen ==
  dataIn : Inport
  validIn : Inport  Port=2
  preambleValidIn : Inport  Port=3
  CtrlSigGen : Subsystem
  Delay1 : Delay  DelayLength=1
  Delay10 : Delay  DelayLength=1
  SampleCounter : Subsystem
  SymbolCounter : Subsystem
  pilotGen : Subsystem
  dataOut : Outport  VectorParamsAs1DForOutWhenUnconnected=off
  pilotOut : Outport  Port=2  VectorParamsAs1DForOutWhenUnconnected=off
  pilotEnd : Outport  Port=3  VectorParamsAs1DForOutWhenUnconnected=off
  dataValid : Outport  Port=4  VectorParamsAs1DForOutWhenUnconnected=off
  wires:
  dataIn/1 -> Delay10/1
  Delay10/1 -> dataOut/1
  pilotGen/1(pilOut) -> pilotOut/1
  validIn/1 -> SampleCounter/1(Valid_In), Delay1/1, SymbolCounter/1(ValidIn)
  SymbolCounter/1(Symbl_cnt) -> pilotGen/1(symbCount)
  CtrlSigGen/1(dataValid) -> dataValid/1
  CtrlSigGen/2(pilotEnd) -> pilotEnd/1
  SampleCounter/1(Sample_Cnt) -> CtrlSigGen/2(sampleCount), pilotGen/2(sampleCount)
  Delay1/1 -> CtrlSigGen/1(valid), pilotGen/3(valid)
  preambleValidIn/1 -> SymbolCounter/2(preambleValidIn)

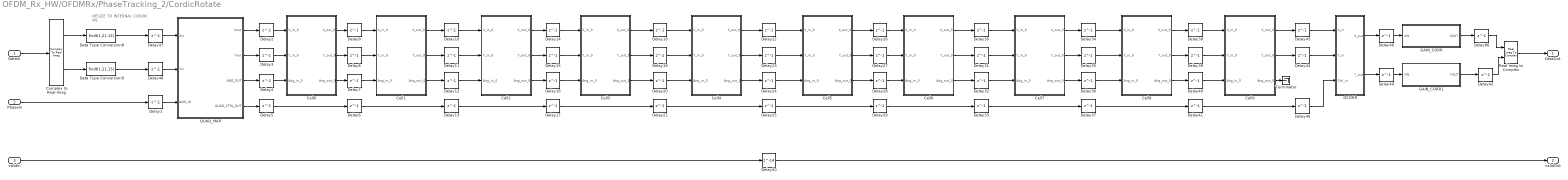
== system OFDM_Rx_HW/OFDMRx/PhaseTracking_2/CordicRotate ==
  note: RESIZE TO INTERNAL
      | CORDIC WL
  DataIn : Inport
  PhaseIn : Inport  Port=2
  validIn : Inport  Port=3
  Cell0 : Subsystem
  Cell1 : Subsystem
  Cell2 : Subsystem
  Cell3 : Subsystem
  Cell4 : Subsystem
  Cell5 : Subsystem
  Cell6 : Subsystem
  Cell7 : Subsystem
  Cell8 : Subsystem
  Cell9 : Subsystem
  Complex to Real-Imag : ComplexToRealImag
  Data Type Conversion8 : DataTypeConversion  OutDataTypeStr=fixdt(1,21,15)
  Data Type Conversion9 : DataTypeConversion  OutDataTypeStr=fixdt(1,21,15)
  Delay{1..49,86} (50 alike) : Delay  DelayLength=1
  Delay50 : Delay  DelayLength=14
  GAIN_CORR : Subsystem
  GAIN_CORR1 : Subsystem
  QCORR : Subsystem
  QUAD_MAP : Subsystem
  Real-Imag to Complex : RealImagToComplex
  Terminator : Terminator
  "DataOut  " : Outport  VectorParamsAs1DForOutWhenUnconnected=off
  validOut : Outport  Port=2  VectorParamsAs1DForOutWhenUnconnected=off
  wires:
  QCORR/1(X_out) -> Delay46/1
  PhaseIn/1 -> Delay1/1
  Data Type Conversion9/1 -> Delay48/1
  Data Type Conversion8/1 -> Delay47/1
  Delay45/1 -> QCORR/3(Ctrl_in)
  Delay4/1 -> Cell0/3(Ang_in_0)
  Delay1/1 -> QUAD_MAP/3(ANG_IN)
  QCORR/2(Y_out) -> Delay49/1
  Delay49/1 -> GAIN_CORR1/1(YIN)
  Delay46/1 -> GAIN_CORR/1(XIN)
  Delay44/1 -> QCORR/2(Y_in)
  Delay43/1 -> QCORR/1(X_in)
  Cell9/2(Y_out_0) -> Delay44/1
  Cell9/1(X_out_0) -> Delay43/1
  Delay41/1 -> Delay45/1
  Cell9/3(Ang_out_0) -> Terminator/1
  GAIN_CORR1/1(YOUT) -> Delay42/1
  Cell8/1(X_out_0) -> Delay38/1
  Cell8/2(Y_out_0) -> Delay39/1
  Cell8/3(Ang_out_0) -> Delay40/1
  Delay37/1 -> Delay41/1
  Delay38/1 -> Cell9/1(X_in_0)
  Delay39/1 -> Cell9/2(Y_in_0)
  Delay40/1 -> Cell9/3(Ang_in_0)
  Delay36/1 -> Cell8/3(Ang_in_0)
  Delay35/1 -> Cell8/2(Y_in_0)
  Delay34/1 -> Cell8/1(X_in_0)
  Delay33/1 -> Delay37/1
  Cell7/3(Ang_out_0) -> Delay36/1
  Cell7/2(Y_out_0) -> Delay35/1
  Cell7/1(X_out_0) -> Delay34/1
  Cell6/1(X_out_0) -> Delay30/1
  Cell6/2(Y_out_0) -> Delay31/1
  Cell6/3(Ang_out_0) -> Delay32/1
  Delay29/1 -> Delay33/1
  Delay30/1 -> Cell7/1(X_in_0)
  Delay31/1 -> Cell7/2(Y_in_0)
  Delay32/1 -> Cell7/3(Ang_in_0)
  Delay28/1 -> Cell6/3(Ang_in_0)
  Delay27/1 -> Cell6/2(Y_in_0)
  Delay26/1 -> Cell6/1(X_in_0)
  Delay25/1 -> Delay29/1
  Cell5/3(Ang_out_0) -> Delay28/1
  Cell5/2(Y_out_0) -> Delay27/1
  Cell5/1(X_out_0) -> Delay26/1
  Cell4/1(X_out_0) -> Delay22/1
  Cell4/2(Y_out_0) -> Delay23/1
  Cell4/3(Ang_out_0) -> Delay24/1
  Delay21/1 -> Delay25/1
  Delay22/1 -> Cell5/1(X_in_0)
  Delay23/1 -> Cell5/2(Y_in_0)
  Delay24/1 -> Cell5/3(Ang_in_0)
  Delay20/1 -> Cell4/3(Ang_in_0)
  Delay19/1 -> Cell4/2(Y_in_0)
  Delay18/1 -> Cell4/1(X_in_0)
  Delay17/1 -> Delay21/1
  Cell3/3(Ang_out_0) -> Delay20/1
  Cell3/2(Y_out_0) -> Delay19/1
  Cell3/1(X_out_0) -> Delay18/1
  Cell2/1(X_out_0) -> Delay14/1
  Cell2/2(Y_out_0) -> Delay15/1
  Cell2/3(Ang_out_0) -> Delay16/1
  Delay13/1 -> Delay17/1
  Delay14/1 -> Cell3/1(X_in_0)
  Delay15/1 -> Cell3/2(Y_in_0)
  Delay16/1 -> Cell3/3(Ang_in_0)
  Delay12/1 -> Cell2/3(Ang_in_0)
  Delay11/1 -> Cell2/2(Y_in_0)
  Delay10/1 -> Cell2/1(X_in_0)
  Delay6/1 -> Delay13/1
  Cell1/3(Ang_out_0) -> Delay12/1
  Cell1/2(Y_out_0) -> Delay11/1
  Cell1/1(X_out_0) -> Delay10/1
  Delay9/1 -> Cell1/1(X_in_0)
  Delay8/1 -> Cell1/2(Y_in_0)
  Delay7/1 -> Cell1/3(Ang_in_0)
  Delay5/1 -> Delay6/1
  Cell0/3(Ang_out_0) -> Delay7/1
  Cell0/2(Y_out_0) -> Delay8/1
  Cell0/1(X_out_0) -> Delay9/1
  QUAD_MAP/4(QUAD_CTRL_OUT) -> Delay5/1
  Delay3/1 -> Cell0/2(Y_in_0)
  Delay2/1 -> Cell0/1(X_in_0)
  QUAD_MAP/3(ANG_OUT) -> Delay4/1
  QUAD_MAP/2(Yout) -> Delay3/1
  QUAD_MAP/1(Xout) -> Delay2/1
  Delay47/1 -> QUAD_MAP/1(Xin)
  Delay48/1 -> QUAD_MAP/2(Yin)
  GAIN_CORR/1(XOUT) -> Delay86/1
  Complex to Real-Imag/2 -> Data Type Conversion9/1
  DataIn/1 -> Complex to Real-Imag/1
  Complex to Real-Imag/1 -> Data Type Conversion8/1
  Delay86/1 -> Real-Imag to Complex/1
  Delay42/1 -> Real-Imag to Complex/2
  Real-Imag to Complex/1 -> "DataOut  "/1
  validIn/1 -> Delay50/1
  Delay50/1 -> validOut/1

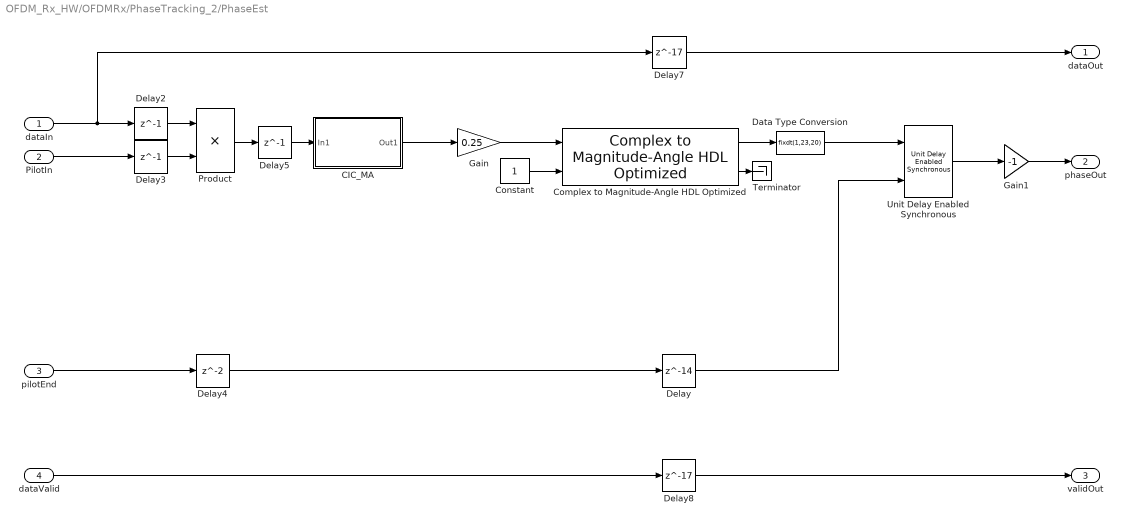
== system OFDM_Rx_HW/OFDMRx/PhaseTracking_2/PhaseEst ==
  dataIn : Inport
  PilotIn : Inport  Port=2
  pilotEnd : Inport  Port=3
  dataValid : Inport  Port=4
  CIC_MA : Subsystem
  Complex to Magnitude-Angle HDL Optimized : dsphdlmathfun/Complex to Magnitude-Angle HDL Optimized  NumIterationsSource=Property  NumIterations=10  OutputFormat=Angle  AngleFormat=Radians  ScaleOutput=off  SimulateUsing=Code generation
      settings: SourceProductBaseCode=DS
  Constant : Constant  OutDataTypeStr=boolean  SampleTime=1/fs
  Data Type Conversion : DataTypeConversion  OutDataTypeStr=fixdt(1,23,20)
  Delay : Delay  DelayLength=14
  Delay2 : Delay  DelayLength=1
  Delay3 : Delay  DelayLength=1
  Delay4 : Delay
  Delay5 : Delay  DelayLength=1
  Delay7 : Delay  DelayLength=17
  Delay8 : Delay  DelayLength=17
  Gain : Gain  Gain=0.25  OutDataTypeStr=fixdt(1,18,15)
  Gain1 : Gain  Gain=-1  OutDataTypeStr=fixdt(1,23,20)
  Product : Product  OutDataTypeStr=fixdt(1,18,15)
  Terminator : Terminator
  Unit Delay Enabled Synchronous : hdlsllib/Discrete/Unit Delay Enabled Synchronous  InitialCondition=0.0  SampleTime=-1
      settings: SourceProductBaseCode=SL
  dataOut : Outport  VectorParamsAs1DForOutWhenUnconnected=off
  phaseOut : Outport  Port=2  VectorParamsAs1DForOutWhenUnconnected=off
  validOut : Outport  Port=3  VectorParamsAs1DForOutWhenUnconnected=off
  wires:
  CIC_MA/1(Out1) -> Gain/1
  Delay/1 -> Unit Delay Enabled Synchronous/2
  PilotIn/1 -> Delay3/1
  dataIn/1 -> Delay7/1, Delay2/1
  Product/1 -> Delay5/1
  Delay2/1 -> Product/1
  Delay3/1 -> Product/2
  Delay5/1 -> CIC_MA/1(In1)
  pilotEnd/1 -> Delay4/1
  dataValid/1 -> Delay8/1
  Delay7/1 -> dataOut/1
  Unit Delay Enabled Synchronous/1 -> Gain1/1
  Delay8/1 -> validOut/1
  Constant/1 -> Complex to Magnitude-Angle HDL Optimized/2
  Gain/1 -> Complex to Magnitude-Angle HDL Optimized/1
  Complex to Magnitude-Angle HDL Optimized/1 -> Data Type Conversion/1
  Complex to Magnitude-Angle HDL Optimized/2 -> Terminator/1
  Delay4/1 -> Delay/1
  Gain1/1 -> phaseOut/1
  Data Type Conversion/1 -> Unit Delay Enabled Synchronous/1

== system OFDM_Rx_HW/OFDMRx/PhaseTracking_2/PilotCtrlGen ==
  dataIn : Inport
  ValidIn : Inport  Port=2
  preambleValidIn : Inport  Port=3
  CtrlSigGen : Subsystem
  Delay1 : Delay  DelayLength=1
  Delay10 : Delay  DelayLength=1
  SampleCounter : Subsystem
  SymbolCounter : Subsystem
  pilotGen : Subsystem
  dataOut : Outport  VectorParamsAs1DForOutWhenUnconnected=off
  pilotOut : Outport  Port=2  VectorParamsAs1DForOutWhenUnconnected=off
  PilotEnd : Outport  Port=3  VectorParamsAs1DForOutWhenUnconnected=off
  dataValid : Outport  Port=4  VectorParamsAs1DForOutWhenUnconnected=off
  wires:
  dataIn/1 -> Delay10/1
  Delay10/1 -> dataOut/1
  pilotGen/1(pilOut) -> pilotOut/1
  ValidIn/1 -> Delay1/1, SampleCounter/1(Valid_In), SymbolCounter/1(ValidIn)
  SymbolCounter/1(Symbl_cnt) -> pilotGen/1(symbCount)
  CtrlSigGen/1(dataValid) -> dataValid/1
  CtrlSigGen/2(pilotEnd) -> PilotEnd/1
  SampleCounter/1(Sample_Cnt) -> CtrlSigGen/2(sampleCount), pilotGen/2(sampleCount)
  Delay1/1 -> CtrlSigGen/1(valid), pilotGen/3(valid)
  preambleValidIn/1 -> SymbolCounter/2(preambleValidIn)

== system OFDM_Rx_HW/OFDMRx/Synchronisation/CoarseFreqCorr ==
  note: Generate complex sinusoid with a frequency equal
      | to the estimated frequency offset.
  note: Correct frequency offset
  note: Reccord the phase of the averaged autocorrelation at the coarse
      | timing point.
  dataIn : Inport
  frameDet : Inport  Port=2
  phaseIn : Inport  Port=3
  Constant : Constant  VectorParams1D=off  OutDataTypeStr=boolean  SampleTime=1/fs
  Delay{,2,5,7} (4 alike) : Delay  DelayLength=1
  Delay1 : Delay  DelayLength=9
  Delay3 : Delay  DelayLength=6
  Gain : Gain  Gain=2048  OutDataTypeStr=uint16
  Math Function : Math  Operator=conj  SignedPower=on  RndMeth=Zero  SaturateOnIntegerOverflow=on
  NCO HDL Optimized : dsphdlsigops/NCO HDL Optimized  PhaseIncrementSource=Input port  PhaseIncrement=100  PhaseOffsetSource=Property  PhaseOffset=0  DitherSource=Property  NumDitherBits=4  SamplesPerFrame=1  LUTCompress=on  ResetAction=off  Waveform=Complex exponential  PhasePort=off  SimulateUsing=Code generation  AccumulatorWL=16  PhaseQuantization=on  NumQuantizerAccumulatorBits=12  OutputDataType=Binary point scaling  OutputWL=16  OutputFL=14
      settings: SourceProductBaseCode=DS
  Product : Product  OutDataTypeStr=fixdt(1,16,14)
  RsingEdge : Subsystem
  Terminator : Terminator
  Unit Delay Enabled Synchronous : hdlsllib/Discrete/Unit Delay Enabled Synchronous  InitialCondition=0.0  SampleTime=-1
      settings: SourceProductBaseCode=SL
  dataOut : Outport  VectorParamsAs1DForOutWhenUnconnected=off
  frameDetOut : Outport  Port=2  VectorParamsAs1DForOutWhenUnconnected=off
  wires:
  Constant/1 -> NCO HDL Optimized/2
  NCO HDL Optimized/2 -> Terminator/1
  NCO HDL Optimized/1 -> Math Function/1
  Gain/1 -> NCO HDL Optimized/1
  Unit Delay Enabled Synchronous/1 -> Gain/1
  Delay2/1 -> Delay3/1
  frameDet/1 -> RsingEdge/1(In1), Delay1/1
  RsingEdge/1(Out1) -> Unit Delay Enabled Synchronous/2
  phaseIn/1 -> Unit Delay Enabled Synchronous/1
  dataIn/1 -> Delay2/1
  Delay/1 -> Product/1
  Delay5/1 -> Product/2
  Product/1 -> Delay7/1
  Delay3/1 -> Delay/1
  Math Function/1 -> Delay5/1
  Delay1/1 -> frameDetOut/1
  Delay7/1 -> dataOut/1

== system OFDM_Rx_HW/OFDMRx/Synchronisation/ControlSigGen ==
  validIn : Inport
  OR : Logic  Operator=OR  IconShape=distinctive  AllPortsSameDT=off  OutDataTypeStr=boolean
  PreambleValidGen : Subsystem
  dataValidGen : Subsystem
  FFTValid : Outport  VectorParamsAs1DForOutWhenUnconnected=off
  dataValid : Outport  Port=2  VectorParamsAs1DForOutWhenUnconnected=off
  preambleValid : Outport  Port=3  VectorParamsAs1DForOutWhenUnconnected=off
  wires:
  validIn/1 -> dataValidGen/2(enb1), PreambleValidGen/1(ValidIn)
  PreambleValidGen/1(y) -> preambleValid/1, OR/1, dataValidGen/1(enb)
  dataValidGen/1(y) -> OR/2, dataValid/1
  OR/1 -> FFTValid/1

== system OFDM_Rx_HW/OFDMRx/Synchronisation/Delay ==
  note: Delay coarse timing point from middle of L-STF
      | to beginning of 1st repetition of L-LTF
  data : Inport
  strobe : Inport  Port=2
  Delay3 : Delay  DelayLength=108  InputProcessing=Columns as channels (frame based)
  dataOut : Outport
  strobeOut : Outport  Port=2
  wires:
  strobe/1 -> Delay3/1
  Delay3/1 -> strobeOut/1
  data/1 -> dataOut/1

== system OFDM_Rx_HW/OFDMRx/Synchronisation/FrameDetect ==
  note: The frame is detected when the timing metric exceeds the threshold for 30 successive samples. This
      | corresponds to the coarse timing point, which should occur in the middle of the L-STF.
  leftIn : Inport
  rightIn : Inport  Port=2
  phaseIn : Inport  Port=3
  Compare To Constant : simulink/Logic and Bit Operations/Compare To Constant  relop===  const=29  OutDataTypeStr=boolean
  Delay{,2..4} (4 alike) : Delay  DelayLength=1
  Frame Detection Valid Gen : Subsystem
  HDL Counter : hdlsllib/Sources/HDL Counter  CountType=Count limited  CountInit=0  CountStep=1  CountMax=29  CountFromType=Initial value  CountFrom=0  CountResetPort=on  CountLoadPort=off  CountEnbPort=on  CountDirPort=off  CountDataType=Unsigned  CountWordLen=5  CountFracLen=0  CountSampTime=1
  Logical Operator : Logic  Operator=OR  IconShape=distinctive  AllPortsSameDT=off  OutDataTypeStr=boolean
  Logical Operator1 : Logic  Operator=NOT  IconShape=distinctive  AllPortsSameDT=off  OutDataTypeStr=boolean
  Relational Operator : RelationalOperator  Operator=>  OutDataTypeStr=boolean  RndMeth=Simplest
  frameDet : Outport  VectorParamsAs1DForOutWhenUnconnected=off
  phaseOut : Outport  Port=2  VectorParamsAs1DForOutWhenUnconnected=off
  wires:
  Delay4/1 -> Delay/1
  Delay2/1 -> Relational Operator/1
  Frame Detection Valid Gen/1(frameDet) -> frameDet/1
  Delay/1 -> phaseOut/1
  leftIn/1 -> Delay2/1
  phaseIn/1 -> Delay4/1
  Logical Operator/1 -> HDL Counter/1
  Compare To Constant/1 -> Logical Operator/1, Frame Detection Valid Gen/1(enable)
  HDL Counter/1 -> Compare To Constant/1
  rightIn/1 -> Delay3/1
  Logical Operator1/1 -> Logical Operator/2
  Relational Operator/1 -> Logical Operator1/1, HDL Counter/2
  Delay3/1 -> Relational Operator/2

== system OFDM_Rx_HW/OFDMRx/Synchronisation/SchmidlCoxMetric  ==
  note: (R(d))^2 x thresh
  note: |P(d)|^2
  note: The Schmidl & Cox timing metric is used for frame detection. The timing metric, M(d), is compared to a threshold
      | to determine if a frame is present. In order to avoid division, we re-arrange the timing metric as |P(d)|^2 > (R(d))^2 x thresh.
      | The phase of the averaged autocorrelation is also determined for Carrier Frequency Offset (CFO) estimation purposes.
  dataIn : Inport
  threshold : Inport  Port=2
  Abs2 : Subsystem
  AutoCorr : Subsystem
  CIC_ma : Subsystem
  CIC_ma1 : Subsystem
  Data Type Conversion : DataTypeConversion  OutDataTypeStr=fixdt(0,32,31)  ConvertRealWorld=Stored Integer (SI)
  Delay : Delay  DelayLength=14
  Delay2 : Delay
  MagPhase : Subsystem
  Sq : Subsystem
  Sq1 : Subsystem
  ThreshMult : Subsystem
  left : Outport  VectorParamsAs1DForOutWhenUnconnected=off
  right : Outport  Port=2  VectorParamsAs1DForOutWhenUnconnected=off
  phase : Outport  Port=3  VectorParamsAs1DForOutWhenUnconnected=off
  wires:
  MagPhase/1(Phase) -> Delay2/1
  Delay2/1 -> phase/1
  CIC_ma/1(Out1) -> MagPhase/1(dataIn)
  AutoCorr/1(AcorrOut) -> CIC_ma/1(In1)
  MagPhase/2(Mag) -> Sq/1(In1)
  Abs2/1(Abs2Out) -> CIC_ma1/1(In1)
  dataIn/1 -> Abs2/1(Abs2In), AutoCorr/1(AcorrIn)
  CIC_ma1/1(Out1) -> Delay/1
  Delay/1 -> Sq1/1(In1)
  Sq1/1(Out1) -> ThreshMult/1(In1)
  ThreshMult/1(Out1) -> right/1
  Sq/1(Out1) -> left/1
  Data Type Conversion/1 -> ThreshMult/2(threshold)
  threshold/1 -> Data Type Conversion/1

== system OFDM_Rx_HW/OFDMRx/ChannelEstEq/ChannelEstimate/ChanEst ==
  note: Store conjugate as this is used in the
      | equaliser.
  note: Read out frequency domain LTS
      | when preamble valid is HIGH and
      | use this to obtain channel estimate.
  note: 1st half
  note: 2nd half
  ChanEstIn : Inport
  PreambValidIn : Inport  Port=2
  Delay : Delay  DelayLength=64
  Delay{1..7} (7 alike) : Delay  DelayLength=1
  Gain : Gain  Gain=0.5  OutDataTypeStr=fixdt(1,17,14)
  HDL Counter : hdlsllib/Sources/HDL Counter  CountType=Count limited  CountInit=0  CountStep=1  CountMax=63  CountFromType=Initial value  CountFrom=0  CountResetPort=off  CountLoadPort=off  CountEnbPort=on  CountDirPort=off  CountDataType=Unsigned  CountWordLen=6  CountFracLen=0  CountSampTime=1
  InvLLTF : Lookup_n-D  NumberOfTableDimensions=1  BreakpointsForDimension1=0:63  IndexSearchMethod=Evenly spaced points  Table=fftshift(LTSfreq)  TableDataTypeStr=fixdt(1,16,0)  InterpMethod=Flat  ExtrapMethod=Clip  DiagnosticForOutOfRangeInput=Error  UseLastTableValue=on  InternalRulePriority=Speed  OutDataTypeStr=fixdt(1,16,0)  RndMeth=Simplest  InputSameDT=on
  Math Function : Math  Operator=conj  SignedPower=on  SaturateOnIntegerOverflow=on
  Product : Product  OutDataTypeStr=fixdt(1,16,14)
  Subtract : Sum
  ChEstOut : Outport  VectorParamsAs1DForOutWhenUnconnected=off
  wires:
  Delay7/1 -> Math Function/1
  Delay6/1 -> Subtract/2, Delay/1
  Delay5/1 -> Product/2
  InvLLTF/1 -> Delay5/1
  Delay4/1 -> Product/1
  HDL Counter/1 -> InvLLTF/1
  Gain/1 -> Delay7/1
  Product/1 -> Delay6/1
  Delay/1 -> Subtract/1
  Math Function/1 -> Delay3/1
  ChanEstIn/1 -> Delay1/1
  PreambValidIn/1 -> Delay2/1
  Delay1/1 -> Delay4/1
  Delay2/1 -> HDL Counter/1
  Delay3/1 -> ChEstOut/1
  Subtract/1 -> Gain/1

== system OFDM_Rx_HW/OFDMRx/ChannelEstEq/ChannelEstimate/WriteEnbAddrGen ==
  In1 : Inport
  AND : Logic  IconShape=distinctive  AllPortsSameDT=off  OutDataTypeStr=boolean
  Compare To Constant : simulink/Logic and Bit Operations/Compare To Constant  relop=>=  const=64  OutDataTypeStr=boolean
  Compare To Constant1 : simulink/Logic and Bit Operations/Compare To Constant  relop=<=  const=127  OutDataTypeStr=boolean
  HDL Counter1 : hdlsllib/Sources/HDL Counter  CountType=Count limited  CountInit=0  CountStep=1  CountMax=63  CountFromType=Initial value  CountFrom=0  CountResetPort=off  CountLoadPort=off  CountEnbPort=on  CountDirPort=off  CountDataType=Unsigned  CountWordLen=6  CountFracLen=0  CountSampTime=1
  HDL Counter2 : hdlsllib/Sources/HDL Counter  CountType=Count limited  CountInit=0  CountStep=1  CountMax=127  CountFromType=Initial value  CountFrom=0  CountResetPort=off  CountLoadPort=off  CountEnbPort=on  CountDirPort=off  CountDataType=Unsigned  CountWordLen=7  CountFracLen=0  CountSampTime=1
  Out1 : Outport  VectorParamsAs1DForOutWhenUnconnected=off
  Out2 : Outport  Port=2  VectorParamsAs1DForOutWhenUnconnected=off
  wires:
  In1/1 -> HDL Counter2/1
  HDL Counter2/1 -> Compare To Constant/1, Compare To Constant1/1
  AND/1 -> Out2/1, HDL Counter1/1
  HDL Counter1/1 -> Out1/1
  Compare To Constant/1 -> AND/1
  Compare To Constant1/1 -> AND/2

== system OFDM_Rx_HW/OFDMRx/ChannelEstEq/Equalise/Abs2 ==
  ChEstIn : Inport
  Add : Sum  OutDataTypeStr=fixdt(0,16,14)
  Complex to Real-Imag : ComplexToRealImag
  Delay{,1..4} (5 alike) : Delay  DelayLength=1
  Product : Product
  Product1 : Product
  Out1 : Outport  VectorParamsAs1DForOutWhenUnconnected=off
  wires:
  Delay3/1 -> Add/2
  Delay2/1 -> Add/1
  Delay1/1 -> Product1/1, Product1/2
  Delay/1 -> Product/2, Product/1
  Complex to Real-Imag/2 -> Delay1/1
  Product1/1 -> Delay3/1
  Product/1 -> Delay2/1
  ChEstIn/1 -> Complex to Real-Imag/1
  Complex to Real-Imag/1 -> Delay/1
  Add/1 -> Delay4/1
  Delay4/1 -> Out1/1

== system OFDM_Rx_HW/OFDMRx/ChannelEstEq/Equalise/Complex Mult ==
  In1 : Inport
  In2 : Inport  Port=2
  Delay4 : Delay  DelayLength=1
  Delay5 : Delay  DelayLength=1
  Delay7 : Delay
  Product1 : Product  OutDataTypeStr=fixdt(1,18,15)
  Out1 : Outport
  wires:
  Product1/1 -> Delay7/1
  Delay4/1 -> Product1/1
  In1/1 -> Delay4/1
  Delay5/1 -> Product1/2
  Delay7/1 -> Out1/1
  In2/1 -> Delay5/1

== system OFDM_Rx_HW/OFDMRx/ChannelEstEq/Equalise/Divide ==
  In1 : Inport
  In2 : Inport  Port=2
  Delay1 : Delay  DelayLength=1
  Delay2 : Delay  DelayLength=1
  Delay8 : Delay  DelayLength=1
  Product2 : Product  OutDataTypeStr=fixdt(1,18,15)
  Reciprocal : Product  Inputs=/  OutDataTypeStr=fixdt(0,25,15)  RndMeth=Zero  SaturateOnIntegerOverflow=on
  dataOutEq : Outport
  wires:
  Reciprocal/1 -> Delay1/1
  In2/1 -> Reciprocal/1
  In1/1 -> Delay8/1
  Delay8/1 -> Product2/1
  Delay1/1 -> Product2/2
  Product2/1 -> Delay2/1
  Delay2/1 -> dataOutEq/1

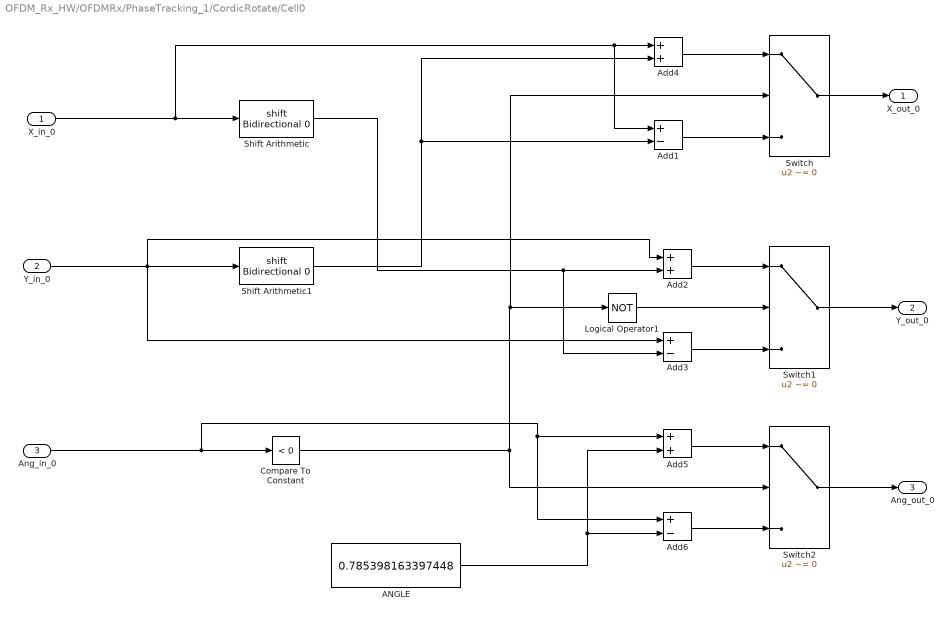
== system OFDM_Rx_HW/OFDMRx/PhaseTracking_1/CordicRotate/Cell0 ==
  X_in_0 : Inport
  Y_in_0 : Inport  Port=2
  Ang_in_0 : Inport  Port=3
  ANGLE : Constant  Value=0.785398163397448  VectorParams1D=off  OutDataTypeStr=fixdt(1,23,20)  SampleTime=1/fs
  Add1 : Sum  Inputs=+-  OutDataTypeStr=fixdt(1,21,15)
  Add2 : Sum  OutDataTypeStr=fixdt(1,21,15)
  Add3 : Sum  Inputs=+-  OutDataTypeStr=fixdt(1,21,15)
  Add4 : Sum  OutDataTypeStr=fixdt(1,21,15)
  Add5 : Sum  OutDataTypeStr=fixdt(1,23,20)
  Add6 : Sum  Inputs=+-  OutDataTypeStr=fixdt(1,23,20)
  Compare To Constant : simulink/Logic and Bit Operations/Compare To Constant  relop=<  const=0  OutDataTypeStr=boolean
  Logical Operator1 : Logic  Operator=NOT  IconShape=distinctive  AllPortsSameDT=off  OutDataTypeStr=boolean
  Shift Arithmetic : ArithShift
  Shift Arithmetic1 : ArithShift
  Switch : Switch  Criteria=u2 ~= 0
  Switch1 : Switch  Criteria=u2 ~= 0
  Switch2 : Switch  Criteria=u2 ~= 0
  X_out_0 : Outport  VectorParamsAs1DForOutWhenUnconnected=off
  Y_out_0 : Outport  Port=2  VectorParamsAs1DForOutWhenUnconnected=off
  Ang_out_0 : Outport  Port=3  VectorParamsAs1DForOutWhenUnconnected=off
  wires:
  ANGLE/1 -> Add5/2, Add6/2
  Logical Operator1/1 -> Switch1/2
  Shift Arithmetic/1 -> Add2/2, Add3/2
  Shift Arithmetic1/1 -> Add4/2, Add1/2
  Compare To Constant/1 -> Switch2/2, Switch/2, Logical Operator1/1
  Ang_in_0/1 -> Compare To Constant/1, Add5/1, Add6/1
  Y_in_0/1 -> Add2/1, Add3/1, Shift Arithmetic1/1
  X_in_0/1 -> Add4/1, Add1/1, Shift Arithmetic/1
  Switch2/1 -> Ang_out_0/1
  Add5/1 -> Switch2/1
  Add6/1 -> Switch2/3
  Switch1/1 -> Y_out_0/1
  Switch/1 -> X_out_0/1
  Add2/1 -> Switch1/1
  Add3/1 -> Switch1/3
  Add1/1 -> Switch/3
  Add4/1 -> Switch/1

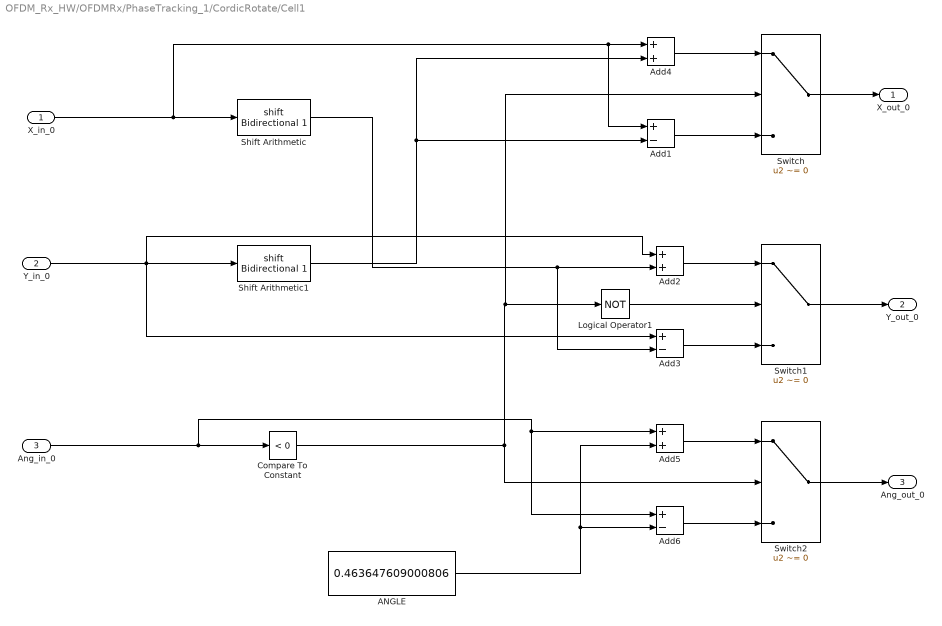
== system OFDM_Rx_HW/OFDMRx/PhaseTracking_1/CordicRotate/Cell1 ==
  X_in_0 : Inport
  Y_in_0 : Inport  Port=2
  Ang_in_0 : Inport  Port=3
  ANGLE : Constant  Value=0.463647609000806  VectorParams1D=off  OutDataTypeStr=fixdt(1,23,20)  SampleTime=1/fs
  Add1 : Sum  Inputs=+-  OutDataTypeStr=fixdt(1,21,15)
  Add2 : Sum  OutDataTypeStr=fixdt(1,21,15)
  Add3 : Sum  Inputs=+-  OutDataTypeStr=fixdt(1,21,15)
  Add4 : Sum  OutDataTypeStr=fixdt(1,21,15)
  Add5 : Sum  OutDataTypeStr=fixdt(1,23,20)
  Add6 : Sum  Inputs=+-  OutDataTypeStr=fixdt(1,23,20)
  Compare To Constant : simulink/Logic and Bit Operations/Compare To Constant  relop=<  const=0  OutDataTypeStr=boolean
  Logical Operator1 : Logic  Operator=NOT  IconShape=distinctive  AllPortsSameDT=off  OutDataTypeStr=boolean
  Shift Arithmetic : ArithShift  BitShiftNumber=1
  Shift Arithmetic1 : ArithShift  BitShiftNumber=1
  Switch : Switch  Criteria=u2 ~= 0
  Switch1 : Switch  Criteria=u2 ~= 0
  Switch2 : Switch  Criteria=u2 ~= 0
  X_out_0 : Outport  VectorParamsAs1DForOutWhenUnconnected=off
  Y_out_0 : Outport  Port=2  VectorParamsAs1DForOutWhenUnconnected=off
  Ang_out_0 : Outport  Port=3  VectorParamsAs1DForOutWhenUnconnected=off
  wires:
  Add4/1 -> Switch/1
  Add1/1 -> Switch/3
  Add3/1 -> Switch1/3
  Add2/1 -> Switch1/1
  Switch/1 -> X_out_0/1
  Switch1/1 -> Y_out_0/1
  Add6/1 -> Switch2/3
  Add5/1 -> Switch2/1
  Switch2/1 -> Ang_out_0/1
  X_in_0/1 -> Shift Arithmetic/1, Add1/1, Add4/1
  Y_in_0/1 -> Shift Arithmetic1/1, Add3/1, Add2/1
  Ang_in_0/1 -> Add6/1, Add5/1, Compare To Constant/1
  Compare To Constant/1 -> Logical Operator1/1, Switch/2, Switch2/2
  Shift Arithmetic1/1 -> Add1/2, Add4/2
  Shift Arithmetic/1 -> Add3/2, Add2/2
  Logical Operator1/1 -> Switch1/2
  ANGLE/1 -> Add6/2, Add5/2
